simulink model "TEST_Live"  (Simulink 8.0)
settings: Solver=ode45  SolverMode=SingleTasking  StartTime=0.0  StopTime=10.0  RelTol=1e-3  AbsTol=1e-6
values from neighbouring files (symbols this model uses):
  IFO = 'L1'    [run_NBtest.m]
  K = 1    [run_NBtest.m]
libraries: cstblocks x3, NbLibrary x3, LiveParts x1
CloseFcn:
  | ;slview('closediagram',bdroot);
settings Model: Creator=controls  LastModifiedBy=ccw  SimulationMode=external  ExtModeTrigMode=oneshot  ExtModeArmWhenConnect=off
settings DataIOCC: LimitDataPoints=off  SignalLoggingSaveFormat=ModelDataLogs
settings OptimizationCC: BlockReduction=off  BooleanDataType=off  ExpressionDepthLimit=128
settings DebuggingCC: SaveWithParameterizedLinksMsg=none  SignalResolutionControl=TryResolveAllWithWarning  SolverPrmCheckMsg=none  MultiTaskDSMMsg=warning  MultiTaskCondExecSysMsg=none  FrameProcessingCompatibilityMsg=error
settings HardwareCC: TargetUnknown=on
settings RTWCC: TemplateMakefile=grt_unix.tmf
settings CodeAppCC: CustomSymbolStrType=$N$R$M_T
settings GRTTargetCC: CodeReplacementLibrary=C89/C90 (ANSI)  CombineOutputUpdateFcns=off  GRTInterface=on

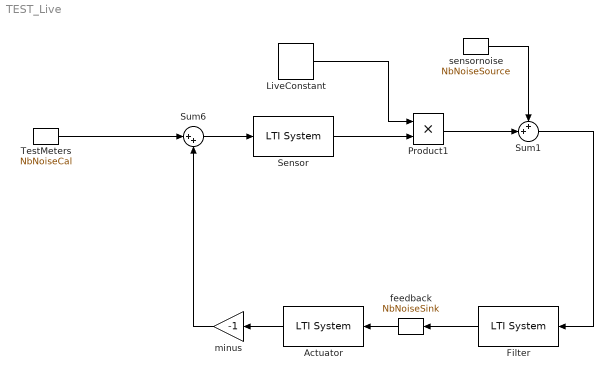
== system TEST_Live ==
  Actuator : cstblocks/LTI System  sys=Act  IC=[]
  Filter : cstblocks/LTI System  sys=Filt  IC=[]
  LiveConstant : LiveParts/LiveConstant  Tag=LiveConstant  K=K  chan=[IFO ':LSC-OMC_DC_GAIN']
      settings: AttributesFormatString=%<Tag>
  Product1 : Product  RndMeth=Zero
  Sensor : cstblocks/LTI System  sys=Sen  IC=[]
  Sum1 : Sum  Inputs=++|
  Sum6 : Sum  Inputs=|++
  TestMeters : NbLibrary/NbNoiseCal  Tag=NbNoiseCal  dof='TST'  unit='displacement [m/rtHz]'
      settings: AttributesFormatString=%<Tag>
  feedback : NbLibrary/NbNoiseSink  Tag=NbNoiseSink  dof='TST'  asd=1  chan=[IFO ':LSC-MC_OUT_DQ']
      settings: AttributesFormatString=%<Tag>
  minus : Gain  Gain=-1
  sensornoise : NbLibrary/NbNoiseSource  Tag=NbNoiseSource  asd=1  chan=''  groupNest=1  group='test noise'  subgroup=''  subsubgroup=''  subsubsubgroup=''
      settings: AttributesFormatString=%<Tag>
  wires:
  Actuator/1 -> minus/1
  TestMeters/1 -> Sum6/1
  Sum6/1 -> Sensor/1
  Sensor/1 -> Product1/2
  LiveConstant/1 -> Product1/1
  feedback/1 -> Actuator/1
  Filter/1 -> feedback/1
  Product1/1 -> Sum1/2
  Sum1/1 -> Filter/1
  sensornoise/1 -> Sum1/1
  minus/1 -> Sum6/2
